simulink model "semi_GSTA"  (R2018b)
(part 5 of 6)

      | 3.11978214555698
      | 3.11690162550175
      | 3.11405076030605
      | 3.11122892447158
      | 3.10843545858463
      | 3.10566971670057
      | 3.10293106378062
      | 3.10021879913599
      | 3.09753244625250
      | 3.09487122390064
      | 3.09223464070947
      | 3.08962203603748
      | 3.08703285163488
      | 3.08446645490365
      | 3.08192232113422
      | 3.07939988891059
      | 3.07689857603428
      | 3.07441784119799
      | 3.07195715319448
      | 3.06951598202208
      | 3.06709380883573
      | 3.06469016924477
      | 3.06230451246091
      | 3.05993638239691
      | 3.05758527826998
      | 3.05525076607482
      | 3.05293240226253
      | 3.05062969114443
      | 3.04834221646154
      | 3.04606956732320
      | 3.04381131969726
      | 3.04156706065192
      | 3.03933642803050
      | 3.03711892963370
      | 3.03491430958135
      | 3.03272210250519
      | 3.03054201726062
      | 3.02837362883845
      | 3.02621666331086
      | 3.02407071095451
      | 3.02193545054863
      | 3.01981061072813
      | 3.01769583511236
      | 3.01559082155978
      | 3.01349524527376
      | 3.01140881468958
      | 3.00933126739202
      | 3.00726228574074
      | 3.00520158099861
      | 3.00314890748047
      | 3.00110392293293
      | 2.99906647456458
      | 2.99703621708606
      | 2.99501289410949
      | 2.99299625459780
      | 2.99098606627627
      | 2.98898203657087
      | 2.98698394801065
      | 2.98499154237256
      | 2.98300460548547
      | 2.98102281553734
      | 2.97904607541363
      | 2.97707396561683
      | 2.97510633519412
      | 2.97314296541241
      | 2.97118359810875
      | 2.96922796716638
      | 2.96727587061390
      | 2.96532702519617
      | 2.96338125575902
      | 2.96143824311458
      | 2.95949775246935
      | 2.95755961486965
      | 2.95562353049714
      | 2.95368923292276
      | 2.95175647570414
      | 2.94982502227136
      | 2.94789457808057
      | 2.94596493387214
      | 2.94403579872125
      | 2.94210692996320
      | 2.94017802086302
      | 2.93824881428972
      | 2.93631897927590
      | 2.93438836749378
      | 2.93245649737284
      | 2.93052324588354
      | 2.92858824308022
      | 2.92665118121399
      | 2.92471177285059
      | 2.92276965818051
      | 2.92082452697233
      | 2.91887614095229
      | 2.91692412711248
      | 2.91496812013002
      | 2.91300775171287
      | 2.91104271704277
      | 2.90907264589652
      | 2.90709714150799
      | 2.90511596140601
      | 2.90312850706189
      | 2.90113458498070
      | 2.89913365170610
      | 2.89712548265997
      | 2.89510946558129
      | 2.89308540675504
      | 2.89105267530287
      | 2.88901091385755
      | 2.88695965093397
      | 2.88489846732708
      | 2.88282689613446
      | 2.88074439951875
      | 2.87865054120751
      | 2.87654475456979
      | 2.87442664057117
      | 2.87229566067561
      | 2.87015117331835
      | 2.86799271407941
      | 2.86581963918398
      | 2.86363148099387
      | 2.86142762220941
      | 2.85920735155886
      | 2.85697020661183
      | 2.85471542876022
      | 2.85244246887728
      | 2.85015058243982
      | 2.84783910621795
      | 2.84550738077758
      | 2.84315454671118
      | 2.84078000339844
      | 2.83838293693869
      | 2.83596252524580
      | 2.83351805785343
      | 2.83104856219340
      | 2.82855336795660
      | 2.82603138903719
      | 2.82348196555058
      | 2.82090396770919
      | 2.81829648659378
      | 2.81565859926631
      | 2.81298921869114
      | 2.81028736604700
      | 2.80755190419153
      | 2.80478179169559
      | 2.80197587467850
      | 2.79913293235327
      | 2.80712830586383
      | 2.82128523630688
      | 2.83525463798016
      | 2.84902194588153
      | 2.86257657927017
      | 2.87591072439296
      | 2.88901853717604
      | 2.90189557633879
      | 2.91453849044498
      | 2.92694458738603
      | 2.93911186559789
      | 2.95103863115482
      | 2.96272357550988
      | 2.97416556565207
      | 2.98536367351372
      | 2.99631709694113
      | 3.00702509153534
      | 3.01748703191344
      | 3.02770223121953
      | 3.03767012351727
      | 3.04739012320962
      | 3.05686159777051
      | 3.06608398301849
      | 3.07505666413517
      | 3.08377902543083
      | 3.09225042123575
      | 3.10047020467985
      | 3.10843771267377
      | 3.11615221464803
      | 3.12361304128435
      | 3.13081943717355
      | 3.13777065833532
      | 3.14446595001287
      | 3.15090450253745
      | 3.15708554754073
      | 3.16300825144826
      | 3.16867177962351
      | 3.17407529079767
      | 3.17921791815645
      | 3.18409879558106
      | 3.18871700295578
      | 3.19307165992376
      | 3.19716186273659
      | 3.20098667670822
      | 3.20454513595059
      | 3.20783634138192
      | 3.21085928487923
      | 3.21361301620209
      | 3.21609658565550
      | 3.21830897933078
      | 3.22024918379920
      | 3.22191623962693
      | 3.22330911513773
      | 3.22442679813585
      | 3.22526829980892
      | 3.22583258398177
      | 3.22611862451515
      | 3.22612545508256
      | 3.22585198674312
      | 3.22529726055747
      | 3.22446024890322
      | 3.22333996481222
      | 3.22193542190961
      | 3.22024565516964
      | 3.21826966283795
      | 3.21600651741966
      | 3.21345532048665
      | 3.21061513133338
      | 3.20748509244790
      | 3.20406435908311
      | 3.20035206141851
      | 3.19634743950864
      | 3.19204974571474
      | 3.18745824967865
      | 3.18257229185982
      | 3.17739124335102
      | 3.17191453238880
      | 3.16614164179656
      | 3.16007206677337
      | 3.15370548542696
      | 3.14704148147510
      | 3.14007983243745
      | 3.13282036166410
      | 3.12526284923655
      | 3.11740732960465
      | 3.10925384964759
      | 3.10080252817566
      | 3.09205358151413
      | 3.08300731716894
      | 3.07366417816010
      | 3.06402462751530
      | 3.05408936948156
      | 3.04385910699686
      | 3.03333467884214
      | 3.02251704875584
      | 3.01140733261445
      | 3.00000671178170
      | 2.98831655948016
      | 2.97633835240951
      | 2.96407366180765
      | 2.95152424094812
      | 2.93869196750779
      | 2.92557889878555
      | 2.91218712810007
      | 2.89851904343216
      | 2.88457707322019
      | 2.87036386406190
      | 2.85588213629530
      | 2.84113483607283
      | 2.82612498070925
      | 2.81085591444272
      | 2.79533094716306
      | 2.77955366835860
      | 2.76352774472981
      | 2.74725705312867
      | 2.73074559928902
      | 2.71399761954139
      | 2.69701741852612
      | 2.67980950130791
      | 2.66237853672225
      | 2.64472931138953
      | 2.62686677584376
      | 2.60879610870608
      | 2.59052256362495
      | 2.57205152609368
      | 2.55338856269476
      | 2.53453943309432
      | 2.51550991905948
      | 2.49630601506468
      | 2.47693387774956
      | 2.45739972421350
      | 2.43770996008370
      | 2.41787107527671
      | 2.39788967539302
      | 2.37777245552759
      | 2.35752633689803
      | 2.33715819367180
      | 2.31667513500568
      | 2.29608422856774
      | 2.27539272735132
      | 2.25460791649273
      | 2.23373721474488
      | 2.21278806520007
      | 2.19176796705171
      | 2.17068451711264
      | 2.14954528992669
      | 2.12835795664842
      | 2.10713029085454
      | 2.08586999610957
      | 2.06458483731381
      | 2.04328255135115
      | 2.02197098429495
      | 2.00065788617307
      | 1.97935101746045
      | 1.95805823275623
      | 1.93678725226945
      | 1.91554579500365
      | 1.89434156102259
      | 1.87318219503576
      | 1.85207528014097
      | 1.83102846587707
      | 1.81004915716810
      | 1.78914480621793
      | 1.76832275852495
      | 1.74759027002784
      | 1.72695448307366
      | 1.70642255423994
      | 1.68600140676011
      | 1.66569791233751
      | 1.64551881840721
      | 1.62547078399093
      | 1.60556025945008
      | 1.58579365385518
      | 1.56617719391003
      | 1.54671696463145
      | 1.52741891210823
      | 1.50828881277204
      | 1.48933228762263
      | 1.47055476281682
      | 1.45196164702855
      | 1.43355798304179
      | 1.41534871885877
      | 1.39733863092548
      | 1.37953234915520
      | 1.36193418856157
      | 1.34454848130693
      | 1.32737918325795
      | 1.31043015140843
      | 1.29370502102451
      | 1.27720722426033
      | 1.26094000559820
      | 1.24490644146212
      | 1.22910936508236
      | 1.21355144536870
      | 1.19823509938601
      | 1.18316260193811
      | 1.16833600852247
      | 1.15375710543591
      | 1.13942764163600
      | 1.12534901750661
      | 1.11152246409376
      | 1.09794909766575
      | 1.08462977116756
      | 1.07156512866414
      | 1.05875571041400
      | 1.04620179095033
      | 1.03390350201726
      | 1.02186078331722
      | 1.01007336641177
      | 0.998540851146466
      | 0.987262670439364
      | 0.976238054089642
      | 0.965466117424597
      | 0.954945764964108
      | 0.944675736394906
      | 0.934654680003938
      | 0.924881092394557
      | 0.915353274123106
      | 0.906069421281508
      | 0.897027626184382
      | 0.888225812111820
      | 0.879661768085079
      | 0.871333187820497
      | 0.863237727368187
      | 0.855372797935409
      | 0.847735818880622
      | 0.840324062362392
      | 0.833134722897235
      | 0.826164905614775
      | 0.819411683863507
      | 0.812871974164153
      | 0.806542696405188
      | 0.800420685981351
      | 0.794502711754134
      | 0.788785493587930
      | 0.783265759972444
      | 0.777940116793374
      | 0.772805214758613
      | 0.767857593261212
      | 0.763093839587015
      | 0.758510496691734
      | 0.754104133224786
      | 0.749871258087239
      | 0.745808404319114
      | 0.741912115521288
      | 0.738178916762365
      | 0.734605427024746
      | 0.731188157412966
      | 0.727923781807114
      | 0.724808913267417
      | 0.721840209464183
      | 0.719014414838455
      | 0.716328256304180
      | 0.713778569119050
      | 0.711362179324063
      | 0.709076048091099
      | 0.706917117260609
      | 0.704882441379276
      | 0.702969125474347
      | 0.701174322724434
      | 0.699495337170134
      | 0.697929479060775
      | 0.696474150098489
      | 0.695126870479825
      | 0.693885235223881
      | 0.692746905505793
      | 0.691709682616910
      | 0.690771401393235
      | 0.689930034118326
      | 0.689183695425058
      | 0.688530469511740
      | 0.687968683538763
      | 0.687496690703242
      | 0.687113005828351
      | 0.686816202522309
      | 0.686604957243418
      | 0.686478100264523
      | 0.686434555764564
      | 0.686473363498322
      | 0.686593664377185
      | 0.686794678999057
      | 0.687075816761137
      | 0.687436562435366
      | 0.687876423728916
      | 0.688395193033443
      | 0.688992655017827
      | 0.689668709091109
      | 0.690423394469661
      | 0.691256814574132
      | 0.692169268650261
      | 0.693161012569718
      | 0.694232534400044
      | 0.695384403759235
      | 0.696617140180457
      | 0.697931548410722
      | 0.699328470921181
      | 0.700808766280758
      | 0.702373358608575
      | 0.704023393600131
      | 0.705759996397113
      | 0.707584341793691
      | 0.709497713409007
      | 0.711501477643196
      | 0.713596963207095
      | 0.715785705456909
      | 0.718069082024968
      | 0.720448727850176
      | 0.722926116579998
      | 0.725502926498386
      | 0.728180677396296
      | 0.730961049569302
      | 0.733845648343973
      | 0.736836160519296
      | 0.739934123112164
      | 0.743141130366020
      | 0.746458855182837
      | 0.749888807294553
      | 0.753432436028326
      | 0.757091262944662
      | 0.760866600582709
      | 0.764759775960442
      | 0.768772052329176
      | 0.772904486866025
      | 0.777158210616371
      | 0.781534071389423
      | 0.786032870493706
      | 0.790655244186794
      | 0.795401727677358
      | 0.800272564672817
      | 0.805267990778894
      | 0.810387876276408
      | 0.815632002666817
      | 0.820999941448825]
  Mux : Mux  Inputs=6
  Out1 : Outport
  wires:
  1-D Lookup Table4/1 -> Mux/1
  In1/1 -> 1-D Lookup Table4/1, 1-D Lookup Table1/1, 1-D Lookup Table2/1, 1-D Lookup Table5/1, 1-D Lookup Table6/1, 1-D Lookup Table3/1
  Mux/1 -> Out1/1
  1-D Lookup Table1/1 -> Mux/2
  1-D Lookup Table2/1 -> Mux/3
  1-D Lookup Table3/1 -> Mux/4
  1-D Lookup Table5/1 -> Mux/5
  1-D Lookup Table6/1 -> Mux/6
